simulink model "roll_loop"  (Simulink 8.2)
settings: Solver=ode45  StartTime=0.0  StopTime=500  RelTol=1e-3
undefined symbols (not defined in the file): P
settings Model: Creator=paul  LastModifiedBy=paul
settings DataIOCC: SignalLoggingSaveFormat=Dataset
settings OptimizationCC: ExpressionDepthLimit=128
settings DebuggingCC: FcnCallInpInsideContextMsg=EnableAllAsError  StateNameClashWarn=none
settings GRTTargetCC: CombineOutputUpdateFcns=on  GRTInterface=off

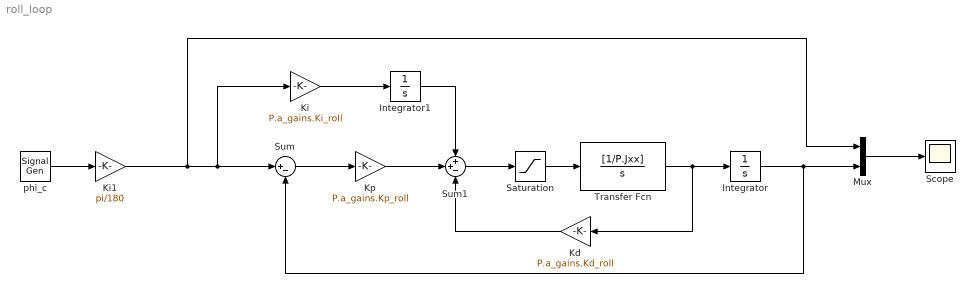
== system roll_loop ==
  Integrator : Integrator
  Integrator1 : Integrator
  Kd : Gain  Gain=P.a_gains.Kd_roll
  Ki : Gain  Gain=P.a_gains.Ki_roll
  Ki1 : Gain  Gain=pi/180
  Kp : Gain  Gain=P.a_gains.Kp_roll
  Mux : Mux  Inputs=2
  Saturation : Saturate  UpperLimit=P.T_phi_max  LowerLimit=-P.T_phi_max
  Scope : Scope
  Sum : Sum  Inputs=|+-
  Sum1 : Sum  Inputs=++-
  Transfer Fcn : TransferFcn  Numerator=[1/P.Jxx]  Denominator=[1 0]
  phi_c : SignalGenerator  WaveForm=square  Amplitude=15  Frequency=0.1  Units=rad/sec
  wires:
  Integrator1/1 -> Sum1/1
  Ki/1 -> Integrator1/1
  Sum/1 -> Kp/1
  Kp/1 -> Sum1/2
  Sum1/1 -> Saturation/1
  Saturation/1 -> Transfer Fcn/1
  Mux/1 -> Scope/1
  phi_c/1 -> Ki1/1
  Kd/1 -> Sum1/3
  Transfer Fcn/1 -> Kd/1, Integrator/1
  Integrator/1 -> Sum/2, Mux/2
  Ki1/1 -> Mux/1, Ki/1, Sum/1
